simulink model "lab1"  (R2019b)
settings: Solver=FixedStepDiscrete  StartTime=0.0  StopTime=150  RelTol=1e-3  EnableMultiTasking=on
settings Model: Creator=s0581533  LastModifiedBy=s0581533

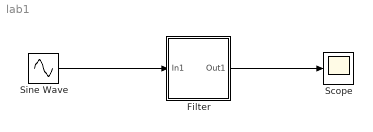
== system lab1 ==
  Filter : Subsystem
  Scope : Scope
  Sine Wave : Sin  Frequency=2*pi*(1/150)  SampleTime=0
  wires:
  Sine Wave/1 -> Filter/1(In1)
  Filter/1(Out1) -> Scope/1

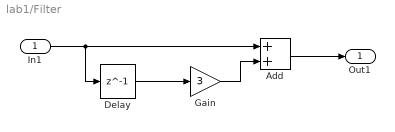
== system lab1/Filter ==
  In1 : Inport
  Add : Sum
  Delay : Delay  DelayLength=1  InitialCondition=0
  Gain : Gain  Gain=3
  Out1 : Outport
  wires:
  In1/1 -> Delay/1, Add/1
  Delay/1 -> Gain/1
  Gain/1 -> Add/2
  Add/1 -> Out1/1
